simulink model "liveness_mc"  (R2021b)
settings: Solver=FixedStepAuto  StartTime=0.0  StopTime=10.0  RelTol=1e-3
undefined symbols (not defined in the file): DiscIntNeverNeededParam, sldvsubsys
libraries: simulink x8, sldvlib x5
settings Model: Creator=marco  LastModifiedBy=angelo
settings ConfigComp: DVMode=PropertyProving  DVTestSuiteOptimization=Auto  DVDetectOutOfBounds=on  DVProvingStrategy=FindViolation  DVModelReferenceHarness=on

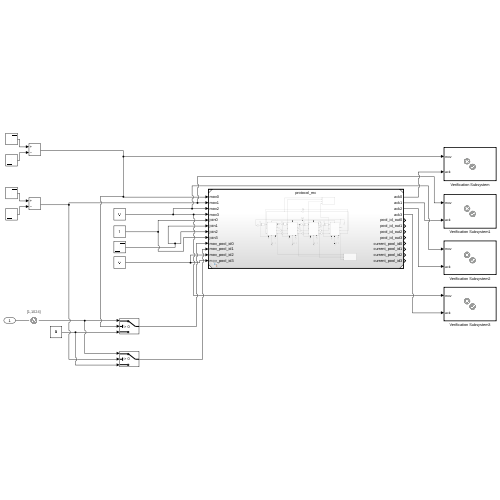
[thumbnail: Simulink's stored preview of the top-level diagram]
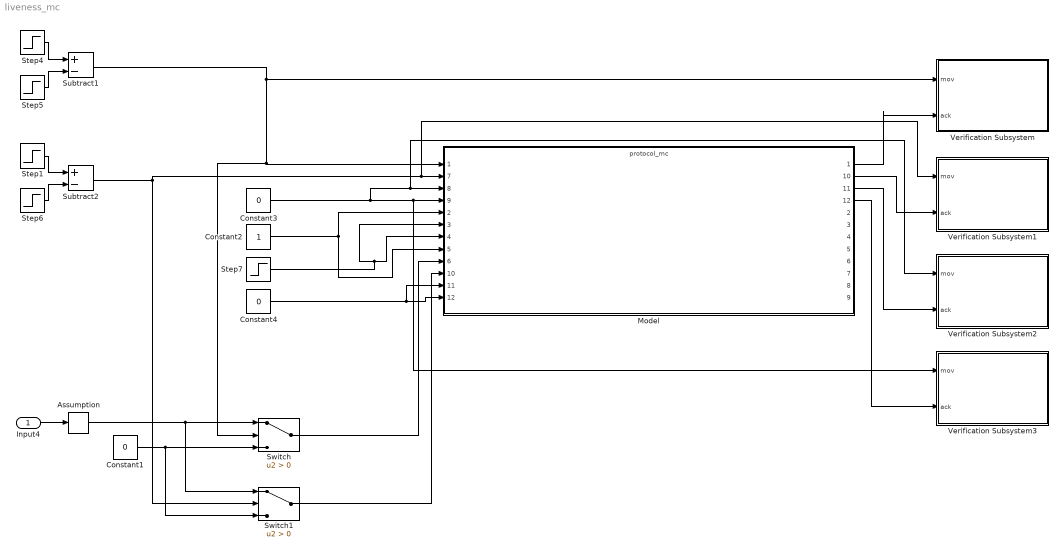
== system liveness_mc ==
  Input4 : Inport  Interpolate=off
  Assumption : sldvlib/Objectives and Constraints/Assumption  enabled=on  customAVTBlockType=Assumption  intervals=[1,1024]  initial=off  dispValues=on  outEnabled=on
      settings: AttributesFormatString=%<intervals>  SourceProductBaseCode=SL
  Constant1 : Constant  Value=0
  Constant2 : Constant
  Constant3 : Constant  Value=0
  Constant4 : Constant  Value=0
  Model : ModelReference  ModelNameDialog=protocol_mc.slx  SimulationMode=Normal  ModelReferenceVersion=1.166
      settings: PortSchema="{\"entries\":[{\"content\":{\"sides\":[{\"content\":{\"connectorIds\":[\"In1\",\"In7\",\"In8\",\"In9\",\"In2\",\"In3\",\"In4\",\"In5\",\"In6\",\"In10\",\"In11\",\"In12\"]},\"type\":\"ConnectorPlacement.EquallySpacedRectSide\",\"uuid\":\"19c3f4b7-089c-465c-b684-d95caf038ffd\"},{\"content\":{\"connectorIds\":[\"Out1\",\"Out10\",\"Out11\",\"Out12\",\"Out2\",\"Out3\",\"Out4\",\"Out5\",\"Out6\",\"Out7\",\"Out8\",\"Out9\"],\"side\":\"RIGHT\"},\"type\":\"ConnectorPlacement.EquallySpacedRectSide\",\"uuid\":\"244a833b-7e56-4340-8fa4-53978e786292\"},{\"content\":{\"connectorIds\":[],\"side\":\"TOP\"},\"type\":\"ConnectorPlacement.EquallySpacedRectSide\",\"uuid\":\"d0116c2f-ddfa-4b0a-ab36-8cec15cb53b1\"}]},\"type\":\"ConnectorPlacement.EquallySpacedConnector\",\"uuid\":\"04a246f8-0c85-4bfe-bf6c-a6795039ecfa\"}],\"packageUris\":[\"http://schema.mathworks.com/mf0/Connector/R2020b\"],\"version\":\"1.0\"}"
  Step1 : Step  Time=3  SampleTime=.2
  Step4 : Step  SampleTime=.2
  Step5 : Step  Time=1.2  SampleTime=.2
  Step6 : Step  Time=3.2  SampleTime=.2
  Step7 : Step  Time=2.2  SampleTime=.2
  Subtract1 : Sum  Inputs=+-
  Subtract2 : Sum  Inputs=+-
  Switch : Switch  Criteria=u2 > Threshold
  Switch1 : Switch  Criteria=u2 > Threshold
  Verification Subsystem : Subsystem  Tag=VerificationSubsystem  DisableCoverage=on  LoadFcn=sldvsubsys('check')  TreatAsAtomicUnit=on  SimViewingDevice=on  mask(VerificationSubsystem){}
      mask init:
      | sldvsubsys('maskInit');
      settings: CopyFcn=sldvsubsys('copy');  OpenFcn=open_system(gcb,'force');
      settings: PreSaveFcn=|
      | set_param(gcb,'SimViewingDevice','on');
      | sldvsubsys('check');
      mask Help: helpview(fullfile(docroot,'toolbox','sldv','sldv.map'),'verificationsubsystem')
      mask Display: image(imread('sldvicon_versubsys.png','BackGroundColor',[1 1 1]),'center');
  Verification Subsystem1 : Subsystem  Tag=VerificationSubsystem  DisableCoverage=on  LoadFcn=sldvsubsys('check')  TreatAsAtomicUnit=on  SimViewingDevice=on  mask(VerificationSubsystem){}
      mask init:
      | sldvsubsys('maskInit');
      settings: CopyFcn=sldvsubsys('copy');  OpenFcn=open_system(gcb,'force');
      settings: PreSaveFcn=|
      | set_param(gcb,'SimViewingDevice','on');
      | sldvsubsys('check');
      mask Help: helpview(fullfile(docroot,'toolbox','sldv','sldv.map'),'verificationsubsystem')
      mask Display: image(imread('sldvicon_versubsys.png','BackGroundColor',[1 1 1]),'center');
  Verification Subsystem2 : Subsystem  Tag=VerificationSubsystem  DisableCoverage=on  LoadFcn=sldvsubsys('check')  TreatAsAtomicUnit=on  SimViewingDevice=on  mask(VerificationSubsystem){}
      mask init:
      | sldvsubsys('maskInit');
      settings: CopyFcn=sldvsubsys('copy');  OpenFcn=open_system(gcb,'force');
      settings: PreSaveFcn=|
      | set_param(gcb,'SimViewingDevice','on');
      | sldvsubsys('check');
      mask Help: helpview(fullfile(docroot,'toolbox','sldv','sldv.map'),'verificationsubsystem')
      mask Display: image(imread('sldvicon_versubsys.png','BackGroundColor',[1 1 1]),'center');
  Verification Subsystem3 : Subsystem  Tag=VerificationSubsystem  DisableCoverage=on  LoadFcn=sldvsubsys('check')  TreatAsAtomicUnit=on  SimViewingDevice=on  mask(VerificationSubsystem){}
      mask init:
      | sldvsubsys('maskInit');
      settings: CopyFcn=sldvsubsys('copy');  OpenFcn=open_system(gcb,'force');
      settings: PreSaveFcn=|
      | set_param(gcb,'SimViewingDevice','on');
      | sldvsubsys('check');
      mask Help: helpview(fullfile(docroot,'toolbox','sldv','sldv.map'),'verificationsubsystem')
      mask Display: image(imread('sldvicon_versubsys.png','BackGroundColor',[1 1 1]),'center');
  wires:
  Model/1 -> Verification Subsystem/2(ack)
  Model/10 -> Verification Subsystem1/2(ack)
  Model/11 -> Verification Subsystem2/2(ack)
  Model/12 -> Verification Subsystem3/2(ack)
  Step6/1 -> Subtract2/2
  Constant2/1 -> Model/5, Model/2
  Switch/1 -> Model/6
  Switch1/1 -> Model/10
  Constant1/1 -> Switch1/3, Switch/3
  Subtract1/1 -> Verification Subsystem/1(mov), Model/1, Switch/2
  Step7/1 -> Model/4, Model/3
  Step4/1 -> Subtract1/1
  Step5/1 -> Subtract1/2
  Input4/1 -> Assumption/1
  Assumption/1 -> Switch1/1, Switch/1
  Step1/1 -> Subtract2/1
  Constant3/1 -> Verification Subsystem3/1(mov), Model/9, Verification Subsystem2/1(mov), Model/8
  Subtract2/1 -> Verification Subsystem1/1(mov), Model/7, Switch1/2
  Constant4/1 -> Model/12, Model/11

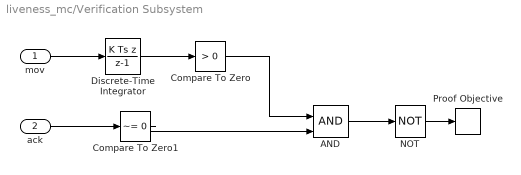
== system liveness_mc/Verification Subsystem ==
  mov : Inport
  ack : Inport  Port=2
  AND : Logic  IconShape=distinctive  AllPortsSameDT=off  OutDataTypeStr=boolean
  Compare To Zero : simulink/Logic and Bit Operations/Compare To Zero  relop=>  OutDataTypeStr=boolean
  Compare To Zero1 : simulink/Logic and Bit Operations/Compare To Zero  relop=~=  OutDataTypeStr=boolean
  Discrete-Time Integrator : DiscreteIntegrator  IntegratorMethod=Integration: Backward Euler  SampleTime=-1  ICPrevOutput=DiscIntNeverNeededParam  ICPrevScaledInput=DiscIntNeverNeededParam
  NOT : Logic  Operator=NOT  IconShape=distinctive  AllPortsSameDT=off  OutDataTypeStr=boolean
  Proof Objective : sldvlib/Objectives and Constraints/Proof Objective  enabled=on  customAVTBlockType=Proof Objective  intervals=true  dispValues=on  outEnabled=off  enableStopSim=off
      settings: AttributesFormatString=%<intervals>  SourceProductBaseCode=SL
  wires:
  Discrete-Time Integrator/1 -> Compare To Zero/1
  mov/1 -> Discrete-Time Integrator/1
  ack/1 -> Compare To Zero1/1
  Compare To Zero/1 -> AND/1
  Compare To Zero1/1 -> AND/2
  AND/1 -> NOT/1
  NOT/1 -> Proof Objective/1

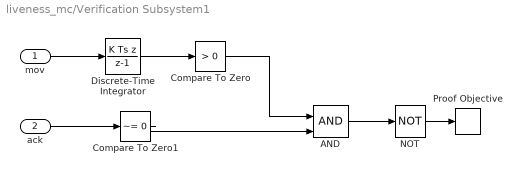
== system liveness_mc/Verification Subsystem1 ==
  mov : Inport
  ack : Inport  Port=2
  AND : Logic  IconShape=distinctive  AllPortsSameDT=off  OutDataTypeStr=boolean
  Compare To Zero : simulink/Logic and Bit Operations/Compare To Zero  relop=>  OutDataTypeStr=boolean
  Compare To Zero1 : simulink/Logic and Bit Operations/Compare To Zero  relop=~=  OutDataTypeStr=boolean
  Discrete-Time Integrator : DiscreteIntegrator  IntegratorMethod=Integration: Backward Euler  SampleTime=-1  ICPrevOutput=DiscIntNeverNeededParam  ICPrevScaledInput=DiscIntNeverNeededParam
  NOT : Logic  Operator=NOT  IconShape=distinctive  AllPortsSameDT=off  OutDataTypeStr=boolean
  Proof Objective : sldvlib/Objectives and Constraints/Proof Objective  enabled=on  customAVTBlockType=Proof Objective  intervals=true  dispValues=on  outEnabled=off  enableStopSim=off
      settings: AttributesFormatString=%<intervals>  SourceProductBaseCode=SL
  wires:
  NOT/1 -> Proof Objective/1
  AND/1 -> NOT/1
  Compare To Zero1/1 -> AND/2
  Compare To Zero/1 -> AND/1
  ack/1 -> Compare To Zero1/1
  mov/1 -> Discrete-Time Integrator/1
  Discrete-Time Integrator/1 -> Compare To Zero/1

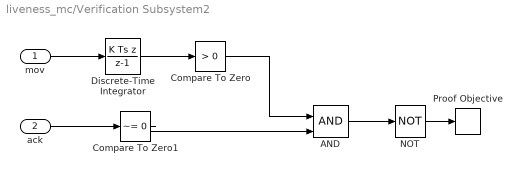
== system liveness_mc/Verification Subsystem2 ==
  mov : Inport
  ack : Inport  Port=2
  AND : Logic  IconShape=distinctive  AllPortsSameDT=off  OutDataTypeStr=boolean
  Compare To Zero : simulink/Logic and Bit Operations/Compare To Zero  relop=>  OutDataTypeStr=boolean
  Compare To Zero1 : simulink/Logic and Bit Operations/Compare To Zero  relop=~=  OutDataTypeStr=boolean
  Discrete-Time Integrator : DiscreteIntegrator  IntegratorMethod=Integration: Backward Euler  SampleTime=-1  ICPrevOutput=DiscIntNeverNeededParam  ICPrevScaledInput=DiscIntNeverNeededParam
  NOT : Logic  Operator=NOT  IconShape=distinctive  AllPortsSameDT=off  OutDataTypeStr=boolean
  Proof Objective : sldvlib/Objectives and Constraints/Proof Objective  enabled=on  customAVTBlockType=Proof Objective  intervals=true  dispValues=on  outEnabled=off  enableStopSim=off
      settings: AttributesFormatString=%<intervals>  SourceProductBaseCode=SL
  wires:
  Discrete-Time Integrator/1 -> Compare To Zero/1
  mov/1 -> Discrete-Time Integrator/1
  ack/1 -> Compare To Zero1/1
  Compare To Zero/1 -> AND/1
  Compare To Zero1/1 -> AND/2
  AND/1 -> NOT/1
  NOT/1 -> Proof Objective/1

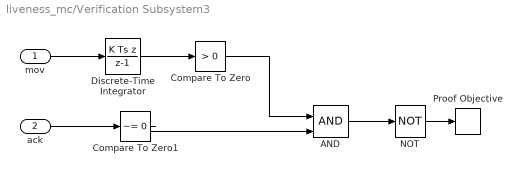
== system liveness_mc/Verification Subsystem3 ==
  mov : Inport
  ack : Inport  Port=2
  AND : Logic  IconShape=distinctive  AllPortsSameDT=off  OutDataTypeStr=boolean
  Compare To Zero : simulink/Logic and Bit Operations/Compare To Zero  relop=>  OutDataTypeStr=boolean
  Compare To Zero1 : simulink/Logic and Bit Operations/Compare To Zero  relop=~=  OutDataTypeStr=boolean
  Discrete-Time Integrator : DiscreteIntegrator  IntegratorMethod=Integration: Backward Euler  SampleTime=-1  ICPrevOutput=DiscIntNeverNeededParam  ICPrevScaledInput=DiscIntNeverNeededParam
  NOT : Logic  Operator=NOT  IconShape=distinctive  AllPortsSameDT=off  OutDataTypeStr=boolean
  Proof Objective : sldvlib/Objectives and Constraints/Proof Objective  enabled=on  customAVTBlockType=Proof Objective  intervals=true  dispValues=on  outEnabled=off  enableStopSim=off
      settings: AttributesFormatString=%<intervals>  SourceProductBaseCode=SL
  wires:
  NOT/1 -> Proof Objective/1
  AND/1 -> NOT/1
  Compare To Zero1/1 -> AND/2
  Compare To Zero/1 -> AND/1
  ack/1 -> Compare To Zero1/1
  mov/1 -> Discrete-Time Integrator/1
  Discrete-Time Integrator/1 -> Compare To Zero/1
